simulink model "iface2"  (R2018b)
settings: Solver=FixedStepDiscrete  StartTime=0.0  StopTime=10.0  RelTol=1e-3
undefined symbols (not defined in the file): myBool, myInteger, myReal, mySeqOfVar
settings Model: Creator=matlab  LastModifiedBy=matlab
settings DataIOCC: SaveOutput=off  SignalLogging=off  SaveTime=off
settings OptimizationCC: DefaultParameterBehavior=Inlined  EnhancedBackFolding=on  PassReuseOutputArgsAs=Individual arguments  OptimizeBlockOrder=speed  DifferentSizesBufferReuse=on  OptimizationCustomize=off
settings DebuggingCC: ParameterTunabilityLossMsg=error
settings SFSimCC: MATLABDynamicMemAlloc=off
settings RTWCC: SystemTargetFile=ert.tlc  TemplateMakefile=ert_default_tmf  PostCodeGenCommand=packNGo(buildInfo);  GenerateReport=on  IncludeHyperlinkInReport=on  LaunchReport=on  GenerateTraceInfo=on  GenerateTraceReport=on  GenerateTraceReportSl=on  GenerateTraceReportSf=on  GenerateTraceReportEml=on
settings CodeAppCC: ForceParamTrailComments=on  IgnoreCustomStorageClasses=off  OperatorAnnotations=on  SimulinkDataObjDesc=on  SFDataObjDesc=on  InsertBlockDesc=on
settings ERTTargetCC: TargetLangStandard=C99 (ISO)  GenerateSampleERTMain=on  InlinedParameterPlacement=NonHierarchical  ERTCustomFileTemplate=example_file_process.tlc

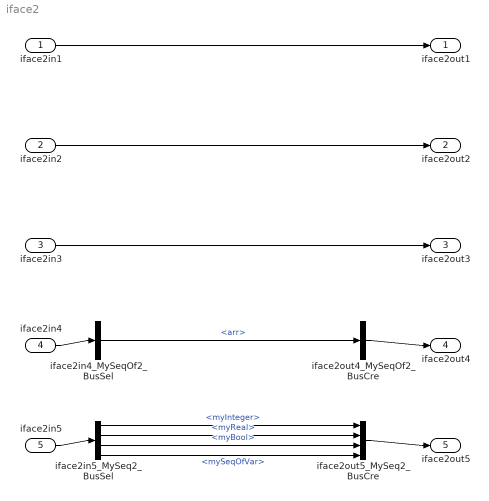
== system iface2 ==
  iface2in1 : Inport  OutDataTypeStr=MyInteger2  BusOutputAsStruct=on
  iface2in2 : Inport  Port=2  OutDataTypeStr=MyReal2  BusOutputAsStruct=on
  iface2in3 : Inport  Port=3  OutDataTypeStr=MyBool2  BusOutputAsStruct=on
  iface2in4 : Inport  Port=4  OutDataTypeStr=Bus: MySeqOf2  BusOutputAsStruct=on
  iface2in5 : Inport  Port=5  OutDataTypeStr=Bus: MySeq2  BusOutputAsStruct=on
  iface2in4_MySeqOf2_BusSel : BusSelector  OutputSignals=arr
  iface2in5_MySeq2_BusSel : BusSelector  OutputSignals=myInteger,myReal,myBool,mySeqOfVar
  iface2out4_MySeqOf2_BusCre : BusCreator  Inputs=1  OutDataTypeStr=Bus: MySeqOf2  NonVirtualBus=on
  iface2out5_MySeq2_BusCre : BusCreator  Inputs=myInteger,myReal,myBool,mySeqOfVar  OutDataTypeStr=Bus: MySeq2  NonVirtualBus=on
  iface2out1 : Outport  OutDataTypeStr=MyInteger2
  iface2out2 : Outport  Port=2  OutDataTypeStr=MyReal2
  iface2out3 : Outport  Port=3  OutDataTypeStr=MyBool2
  iface2out4 : Outport  Port=4  OutDataTypeStr=Bus: MySeqOf2  BusOutputAsStruct=on
  iface2out5 : Outport  Port=5  OutDataTypeStr=Bus: MySeq2  BusOutputAsStruct=on
  wires:
  iface2in4/1 -> iface2in4_MySeqOf2_BusSel/1
  iface2in5/1 -> iface2in5_MySeq2_BusSel/1
  iface2out4_MySeqOf2_BusCre/1 -> iface2out4/1
  iface2out5_MySeq2_BusCre/1 -> iface2out5/1
  iface2in1/1 -> iface2out1/1
  iface2in2/1 -> iface2out2/1
  iface2in3/1 -> iface2out3/1
  iface2in4_MySeqOf2_BusSel/1 -> iface2out4_MySeqOf2_BusCre/1  "<arr>"
  iface2in5_MySeq2_BusSel/1 -> iface2out5_MySeq2_BusCre/1  "<myInteger>"
  iface2in5_MySeq2_BusSel/2 -> iface2out5_MySeq2_BusCre/2  "<myReal>"
  iface2in5_MySeq2_BusSel/3 -> iface2out5_MySeq2_BusCre/3  "<myBool>"
  iface2in5_MySeq2_BusSel/4 -> iface2out5_MySeq2_BusCre/4  "<mySeqOfVar>"
